simulink model "Velo"  (R2019a)
settings: Solver=ode45  StartTime=0  StopTime=4000  FixedStep=1e-3  MaxStep=0.01  RelTol=1e-3  EnableMultiTasking=on
InitFcn:
  | Initialisation
values from neighbouring files (symbols this model uses):
  assist =     [assit_lim.mat]
  cyclist =     [Cyclist_Profile.mat]
  env =     [Uvrier_HEI_Profile.mat]
undefined symbols (not defined in the file or in its folder): cycle
libraries: simulink x1
settings Model: ExtModeTrigMode=oneshot  ExtModeArmWhenConnect=off  Creator=Walter  LastModifiedBy=philippe.barrade
settings DataIOCC: SaveFormat=Array  SignalLoggingSaveFormat=ModelDataLogs  SaveOutput=off  SignalLogging=off  SaveTime=off  ReturnWorkspaceOutputs=off  SignalLoggingName=sigsOut
settings OptimizationCC: BooleanDataType=off  ExpressionDepthLimit=2147483647  InitFltsAndDblsToZero=on  LifeSpan=inf
settings DebuggingCC: SaveWithParameterizedLinksMsg=none  UnderspecifiedInitializationDetection=Classic  MergeDetectMultiDrivingBlocksExec=none  SignalResolutionControl=TryResolveAllWithWarning  MultiTaskDSMMsg=warning  MultiTaskCondExecSysMsg=none  FcnCallInpInsideContextMsg=warning  StateNameClashWarn=warning  SFUnexpectedBacktrackingDiag=warning  SFNoUnconditionalDefaultTransitionDiag=warning  SFExecutionAtInitializationDiag=none  ArithmeticOperatorsInVariantConditions=warning
settings HardwareCC: ProdBitPerPointer=32  ProdBitPerSizeT=32  ProdBitPerPtrDiffT=32  ProdLargestAtomicFloat=None  ProdIntDivRoundTo=Undefined  ProdEndianess=Unspecified  ProdWordSize=32  ProdHWDeviceType=32-bit Generic  TargetUnknown=on
settings ModelReferenceCC: PropagateSignalLabelsOutOfModel=off
settings SFSimCC: SimUseLocalCustomCode=off
settings RTWCC: GenerateMakefile=off  RTWUseLocalCustomCode=off
settings CodeAppCC: StateflowObjectComments=on
settings GRTTargetCC: TargetLangStandard=C89/C90 (ANSI)  ModelReferenceCompliant=off  CompOptLevelCompliant=off  GeneratePreprocessorConditionals=Disable all  CombineOutputUpdateFcns=off  MatFileLogging=off  GRTInterface=on
settings ConfigComp: CovMetricSettings=dw  CovHtmlReporting=on  CovSaveCumulativeToWorkspaceVar=on  CovSaveSingleToWorkspaceVar=on  CovExternalEMLEnable=off  CovSFcnEnable=off

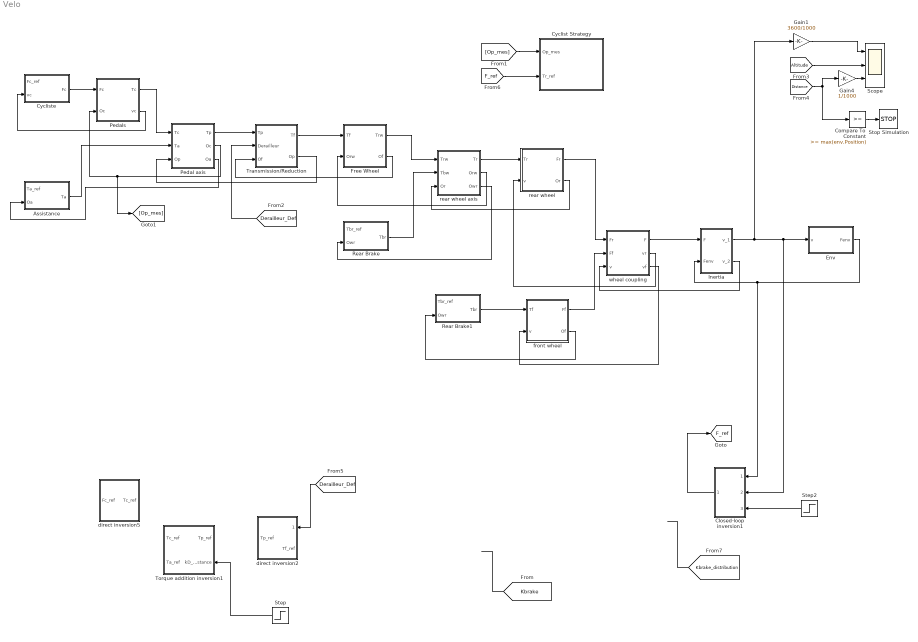
== system Velo ==
  Assistance : Subsystem
      mask Display:
      | plot(0,0,100,100, 1.2*[50,57.68,60.77,63.08,64.97,66.58,68,69.26,70.4, 	71.42,72.36,78.28,80,78.28,72.36,71.42,70.4, 	69.26,68,66.58,64.97,63.08,60.77,57.68,50,42.32, 	39.23,36.92,35.03,33.42,32,30.74,29.6,28.58, 	27.64,21.72,20,21.72,27.64,28.58,29.6,30.74,32, 	33.42,35.03,36.92,39.23,42.32,50]-10, 1.2*[20,21,22,23,24,25,26,27,28,29,30,40,50,60,70,71,72, 	73,74,75,76,77,78,79,80,79,78,77,76,75,74,73,72, 	71,70,60,50,40,30,29,28,27,26,25,24,23,22,21,20]-10)
      | disp('MS')
  Closed-loop inversion1 : Subsystem
      mask Display: plot(0,0,100,100, [10,30,90,70,10,90],[90,10,10,90,90,10])
  Compare To Constant : simulink/Logic and Bit Operations/Compare To Constant  relop=>=  const=max(env.Position)  OutDataTypeStr=boolean
  Cyclist Strategy : Subsystem
      mask Display:
      | color('white');
      | plot(0,0,100,100,[10,30,90,70,10], [90,10,10,90,90]);
  Cycliste : Subsystem
      mask Display:
      | plot(0,0,100,100, 1.2*[50,57.68,60.77,63.08,64.97,66.58,68,69.26,70.4, 	71.42,72.36,78.28,80,78.28,72.36,71.42,70.4, 	69.26,68,66.58,64.97,63.08,60.77,57.68,50,42.32, 	39.23,36.92,35.03,33.42,32,30.74,29.6,28.58, 	27.64,21.72,20,21.72,27.64,28.58,29.6,30.74,32, 	33.42,35.03,36.92,39.23,42.32,50]-10, 1.2*[20,21,22,23,24,25,26,27,28,29,30,40,50,60,70,71,72, 	73,74,75,76,77,78,79,80,79,78,77,76,75,74,73,72, 	71,70,60,50,40,30,29,28,27,26,25,24,23,22,21,20]-10)
      | disp('MS')
  Env : Subsystem
      mask Display:
      | plot(0,0,100,100, 1.2*[50,57.68,60.77,63.08,64.97,66.58,68,69.26,70.4, 	71.42,72.36,78.28,80,78.28,72.36,71.42,70.4, 	69.26,68,66.58,64.97,63.08,60.77,57.68,50,42.32, 	39.23,36.92,35.03,33.42,32,30.74,29.6,28.58, 	27.64,21.72,20,21.72,27.64,28.58,29.6,30.74,32, 	33.42,35.03,36.92,39.23,42.32,50]-10, 1.2*[20,21,22,23,24,25,26,27,28,29,30,40,50,60,70,71,72, 	73,74,75,76,77,78,79,80,79,78,77,76,75,74,73,72, 	71,70,60,50,40,30,29,28,27,26,25,24,23,22,21,20]-10)
      | disp('MS')
  Free Wheel : Subsystem  mask(Hacheur){}
      mask Display: plot(0,0,100,100,[10,10,90,90,10],[90,10,10,90,90])
  Gain1 : Gain  Gain=3600/1000
  Gain4 : Gain  Gain=1/1000
  Inertia : Subsystem  mask(CM){}
      mask Display: plot(0,0,100,100,[10,10,90,90,10],[90,10,10,90,90], [10,90],[10,90])
  Pedal axis : Subsystem  mask(CM){}
      mask Display: plot(0,0,100,100,[35,35,95,95,35],[65,10,10,65,65], [5,5,65,65,5],[90,35,35,90,90])
  Pedals : Subsystem  mask(Hacheur){}
      mask Display: plot(0,0,100,100,[10,10,90,90,10],[90,10,10,90,90])
  Rear Brake : Subsystem
      mask Display:
      | plot(0,0,100,100, 1.2*[50,57.68,60.77,63.08,64.97,66.58,68,69.26,70.4, 	71.42,72.36,78.28,80,78.28,72.36,71.42,70.4, 	69.26,68,66.58,64.97,63.08,60.77,57.68,50,42.32, 	39.23,36.92,35.03,33.42,32,30.74,29.6,28.58, 	27.64,21.72,20,21.72,27.64,28.58,29.6,30.74,32, 	33.42,35.03,36.92,39.23,42.32,50]-10, 1.2*[20,21,22,23,24,25,26,27,28,29,30,40,50,60,70,71,72, 	73,74,75,76,77,78,79,80,79,78,77,76,75,74,73,72, 	71,70,60,50,40,30,29,28,27,26,25,24,23,22,21,20]-10)
      | disp('MS')
  Rear Brake1 : Subsystem
      mask Display:
      | plot(0,0,100,100, 1.2*[50,57.68,60.77,63.08,64.97,66.58,68,69.26,70.4, 	71.42,72.36,78.28,80,78.28,72.36,71.42,70.4, 	69.26,68,66.58,64.97,63.08,60.77,57.68,50,42.32, 	39.23,36.92,35.03,33.42,32,30.74,29.6,28.58, 	27.64,21.72,20,21.72,27.64,28.58,29.6,30.74,32, 	33.42,35.03,36.92,39.23,42.32,50]-10, 1.2*[20,21,22,23,24,25,26,27,28,29,30,40,50,60,70,71,72, 	73,74,75,76,77,78,79,80,79,78,77,76,75,74,73,72, 	71,70,60,50,40,30,29,28,27,26,25,24,23,22,21,20]-10)
      | disp('MS')
  Scope : Scope  NumInputPorts=3
  Step : Step  Time=800  After=0.25  SampleTime=0
  Step2 : Step  Time=5.0  Before=0/3600  After=15000/3600  SampleTime=0
  Stop Simulation : Stop
  Torque addition inversion1 : Subsystem
      mask Display: plot(0,0,100,100,[20,40,100,80,20],[75,20,20,75,75], [0,20,80,60,0],[85,30,30,85,85])
  Transmission/Reduction : Subsystem  mask(Hacheur){}
      mask Display: plot(0,0,100,100,[10,10,90,90,10],[90,10,10,90,90])
  direct inversion2 : Subsystem
      mask Display: plot(0,0,100,100,[10,30,90,70,10],[90,10,10,90,90])
  direct inversion5 : Subsystem
      mask Display: plot(0,0,100,100,[10,30,90,70,10],[90,10,10,90,90])
  front wheel : Subsystem  mask(Hacheur){}
      mask Display: plot(0,0,100,100,[10,10,90,90,10],[90,10,10,90,90])
  rear wheel : Subsystem  mask(Hacheur){}
      mask Display: plot(0,0,100,100,[10,10,90,90,10],[90,10,10,90,90])
  rear wheel axis : Subsystem  mask(CM){}
      mask Display: plot(0,0,100,100,[35,35,95,95,35],[65,10,10,65,65], [5,5,65,65,5],[90,35,35,90,90])
  "wheel coupling " : Subsystem  mask(CM){}
      mask Display: plot(0,0,100,100,[35,35,95,95,35],[65,10,10,65,65], [5,5,65,65,5],[90,35,35,90,90])
  tag scope: F_ref=global
  wires:
  Inertia/1(v_1) -> Gain1/1, Closed-loop inversion1/2(V_mes), Env/1(v)
  Gain1/1 -> Scope/1
  [Altitude] -> Scope/2
  [Distance] -> Compare To Constant/1, Gain4/1
  Gain4/1 -> Scope/3
  [Op_mes] -> Cyclist Strategy/1(Op_mes)
  [F_ref] -> Cyclist Strategy/2(Tr_ref)
  Step/1 -> Torque addition inversion1/2(kD_assistance)
  Compare To Constant/1 -> Stop Simulation/1
  Step2/1 -> Closed-loop inversion1/3(V_ref)
  Cycliste/1(Fc) -> Pedals/1(Fc)
  Pedals/1(Tc) -> Pedal axis/1(Tc)
  Assistance/1(Ta) -> Pedal axis/2(Ta)
  Pedals/2(vc) -> Cycliste/2(vc)
  Pedal axis/2(Oc) -> [Op_mes], Pedals/2(Oc)
  Pedal axis/3(Oa) -> Assistance/2(Oa)
  Pedal axis/1(Tp) -> Transmission/Reduction/1(Tp)
  Transmission/Reduction/1(Tf) -> Free Wheel/1(Tf)
  Free Wheel/1(Trw) -> rear wheel axis/1(Trw)
  Rear Brake/1(Tbr) -> rear wheel axis/2(Tbw)
  Transmission/Reduction/2(Op) -> Pedal axis/3(Op)
  Free Wheel/2(Of) -> Transmission/Reduction/3(Of)
  rear wheel axis/2(Orw) -> Free Wheel/2(Orw)
  rear wheel axis/3(Owr) -> Rear Brake/2(Owr)
  rear wheel axis/1(Tr) -> rear wheel/1(Tr)
  Rear Brake1/1(Tbr) -> front wheel/1(Tf)
  front wheel/2(Of) -> Rear Brake1/2(Owr)
  rear wheel/1(Fr) -> "wheel coupling "/1(Fr)
  front wheel/1(Ff) -> "wheel coupling "/2(Ff)
  "wheel coupling "/2(vr) -> rear wheel/2(v)
  "wheel coupling "/3(vf) -> front wheel/2(v)
  "wheel coupling "/1(F) -> Inertia/1(F)
  Inertia/2(v_2) -> "wheel coupling "/3(v)
  Env/1(Fenv) -> Closed-loop inversion1/1(F_res), Inertia/2(Fenv)
  rear wheel/2(Or) -> rear wheel axis/3(Or)
  Closed-loop inversion1/1(Fr_ref) -> [F_ref]
  [Derailleur_Def] -> Transmission/Reduction/2(Derailleur)
  [Derailleur_Def] -> direct inversion2/1(Derailleur)
  [Kbrake] -> ?
  [Kbrake_distribution] -> ?
  ? -> Cycliste/1(Fc_ref)
  ? -> Assistance/1(Ta_ref)
  ? -> Rear Brake1/1(Tbr_ref)
  ? -> Rear Brake/1(Tbr_ref)

== system Velo/Assistance ==
  Ta_ref : Inport
  Oa : Inport  Port=2
  Memory : Memory
  MinMax : MinMax  Inputs=2
  Ta_lim : Lookup_n-D  NumberOfTableDimensions=1  BreakpointsForDimension1=assist.Op_ref  Table=assist.Ta_lim  InternalRulePriority=Speed  RndMeth=Simplest  InputSameDT=on
  Ta : Outport  InitialOutput=0
  wires:
  Oa/1 -> Memory/1
  Memory/1 -> Ta_lim/1
  MinMax/1 -> Ta/1
  Ta_ref/1 -> MinMax/1
  Ta_lim/1 -> MinMax/2

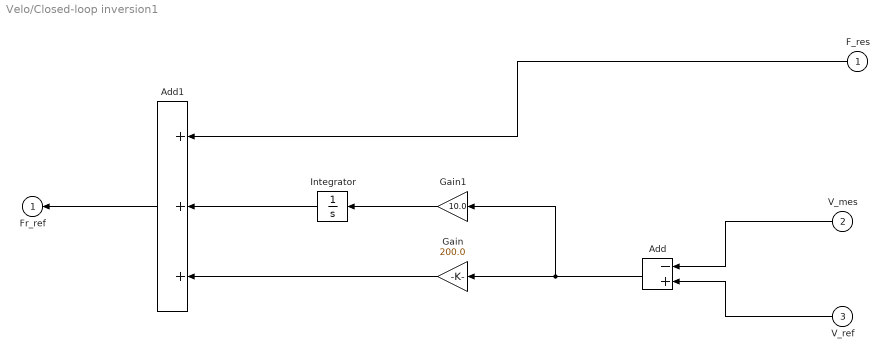
== system Velo/Closed-loop inversion1 ==
  F_res : Inport
  V_mes : Inport  Port=2
  V_ref : Inport  Port=3
  Add : Sum  Inputs=-+
  Add1 : Sum  Inputs=+++
  Gain : Gain  Gain=200.0
  Gain1 : Gain  Gain=10.0
  Integrator : Integrator  LimitOutput=on  UpperSaturationLimit=50  LowerSaturationLimit=-50
  Fr_ref : Outport  InitialOutput=0
  wires:
  V_mes/1 -> Add/1
  Gain1/1 -> Integrator/1
  Add/1 -> Gain1/1, Gain/1
  Add1/1 -> Fr_ref/1
  V_ref/1 -> Add/2
  Gain/1 -> Add1/3
  Integrator/1 -> Add1/2
  F_res/1 -> Add1/1

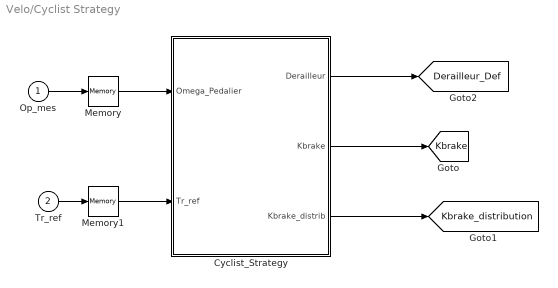
== system Velo/Cyclist Strategy ==
  Op_mes : Inport
  Tr_ref : Inport  Port=2
  Cyclist_Strategy : MATLAB Function  TreatAsAtomicUnit=on
  Memory : Memory
  Memory1 : Memory
  tag scope: Derailleur_Def=global, Kbrake=global, Kbrake_distribution=global
  wires:
  Op_mes/1 -> Memory/1
  Cyclist_Strategy/1(Derailleur) -> [Derailleur_Def]
  Memory/1 -> Cyclist_Strategy/1(Omega_Pedalier)
  Tr_ref/1 -> Memory1/1
  Memory1/1 -> Cyclist_Strategy/2(Tr_ref)
  Cyclist_Strategy/2(Kbrake) -> [Kbrake]
  Cyclist_Strategy/3(Kbrake_distrib) -> [Kbrake_distribution]

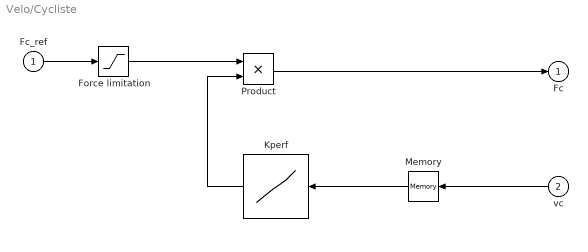
== system Velo/Cycliste ==
  Fc_ref : Inport
  vc : Inport  Port=2
  Force limitation : Saturate  UpperLimit=cyclist.Fc_max
  Kperf : Lookup_n-D  NumberOfTableDimensions=1  BreakpointsForDimension1=cyclist.Vref_ms  Table=cyclist.Kperf  InternalRulePriority=Speed  RndMeth=Simplest  InputSameDT=on
  Memory : Memory
  Product : Product
  Fc : Outport  InitialOutput=0
  wires:
  vc/1 -> Memory/1
  Memory/1 -> Kperf/1
  Product/1 -> Fc/1
  Fc_ref/1 -> Force limitation/1
  Kperf/1 -> Product/2
  Force limitation/1 -> Product/1

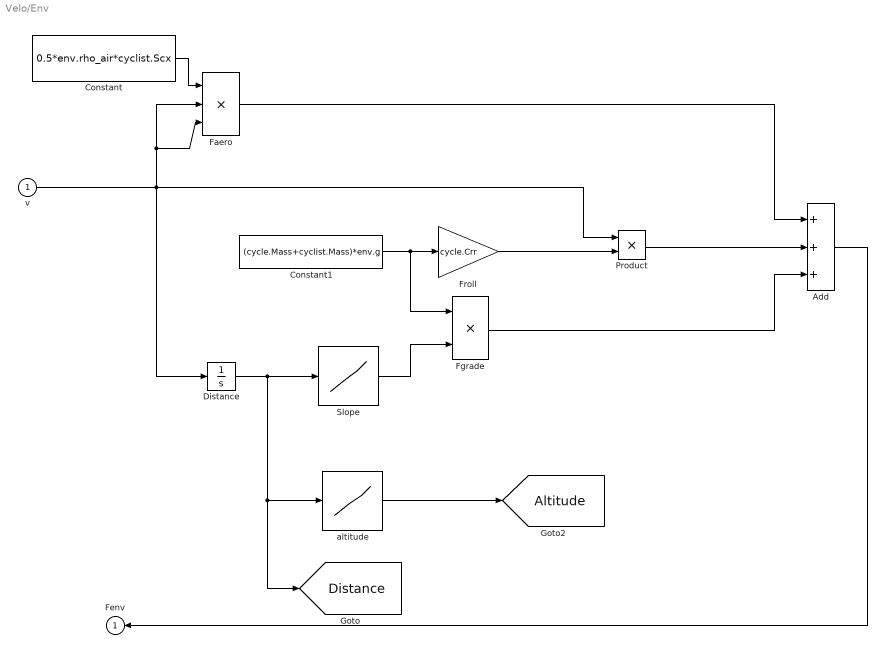
== system Velo/Env ==
  v : Inport
  Add : Sum  Inputs=+++
  Constant : Constant  Value=0.5*env.rho_air*cyclist.Scx
  Constant1 : Constant  Value=(cycle.Mass+cyclist.Mass)*env.g
  Distance : Integrator
  Faero : Product  Inputs=3  RndMeth=Zero
  Fgrade : Product  RndMeth=Zero
  Froll : Gain  Gain=cycle.Crr
  Product : Product  RndMeth=Zero
  Slope : Lookup  InputValues=env.Position  Table=env.Slope  LookUpMeth=Interpolation-Use End Values
  altitude : Lookup  InputValues=env.Position  Table=env.Altitude  LookUpMeth=Interpolation-Use End Values
  Fenv : Outport  InitialOutput=0
  tag scope: Altitude=global, Distance=global
  wires:
  Constant1/1 -> Froll/1, Fgrade/1
  Distance/1 -> [Distance], altitude/1, Slope/1
  Slope/1 -> Fgrade/2
  Faero/1 -> Add/1
  Fgrade/1 -> Add/3
  Add/1 -> Fenv/1
  Product/1 -> Add/2
  Froll/1 -> Product/2
  Constant/1 -> Faero/1
  v/1 -> Product/1, Distance/1, Faero/2, Faero/3
  altitude/1 -> [Altitude]

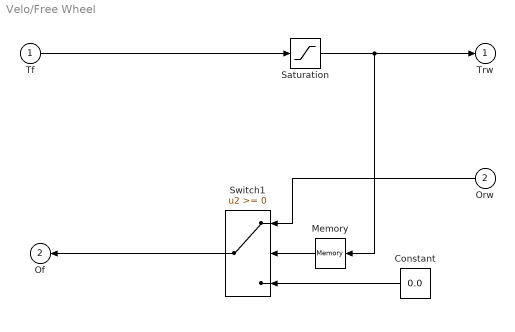
== system Velo/Free Wheel ==
  Tf : Inport
  Orw : Inport  Port=2
  Constant : Constant  Value=0.0
  Memory : Memory
  Saturation : Saturate  UpperLimit=Inf  LowerLimit=-1e-6
  Switch1 : Switch
  Trw : Outport  InitialOutput=0
  Of : Outport  Port=2  InitialOutput=0
  wires:
  Tf/1 -> Saturation/1
  Saturation/1 -> Trw/1, Memory/1
  Orw/1 -> Switch1/1
  Switch1/1 -> Of/1
  Constant/1 -> Switch1/3
  Memory/1 -> Switch1/2

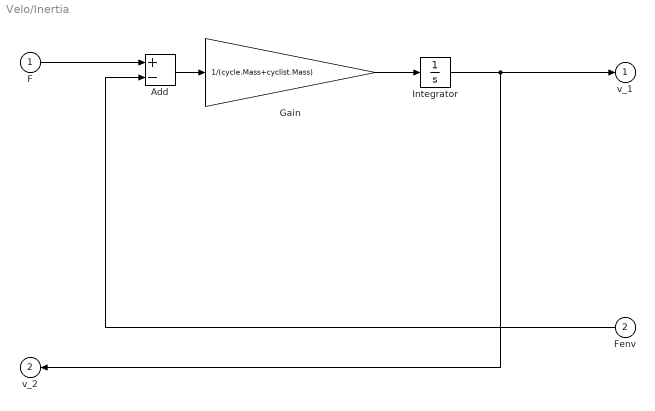
== system Velo/Inertia ==
  F : Inport
  Fenv : Inport  Port=2
  Add : Sum  Inputs=+-
  Gain : Gain  Gain=1/(cycle.Mass+cyclist.Mass)
  Integrator : Integrator
  v_1 : Outport  InitialOutput=0
  v_2 : Outport  Port=2  InitialOutput=0
  wires:
  F/1 -> Add/1
  Fenv/1 -> Add/2
  Add/1 -> Gain/1
  Gain/1 -> Integrator/1
  Integrator/1 -> v_1/1, v_2/1

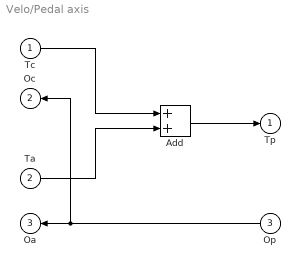
== system Velo/Pedal axis ==
  Tc : Inport
  Ta : Inport  Port=2
  Op : Inport  Port=3
  Add : Sum
  Tp : Outport  InitialOutput=0
  Oc : Outport  Port=2  InitialOutput=0
  Oa : Outport  Port=3  InitialOutput=0
  wires:
  Add/1 -> Tp/1
  Tc/1 -> Add/1
  Ta/1 -> Add/2
  Op/1 -> Oa/1, Oc/1

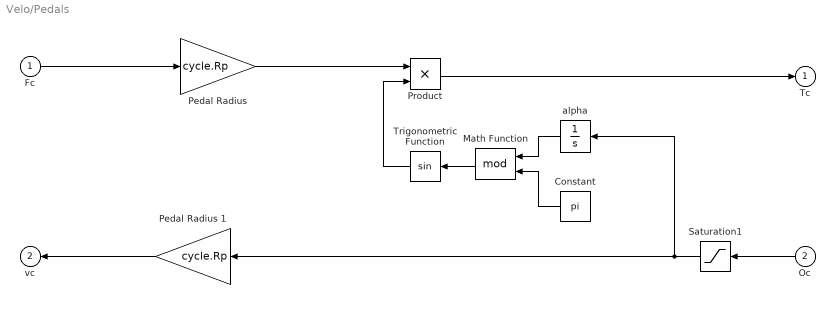
== system Velo/Pedals ==
  Fc : Inport
  Oc : Inport  Port=2
  Constant : Constant  Value=pi
  Math Function : Math  Operator=mod  SaturateOnIntegerOverflow=on
  Pedal Radius : Gain  Gain=cycle.Rp
  Pedal Radius 1 : Gain  Gain=cycle.Rp
  Product : Product
  Saturation1 : Saturate  UpperLimit=Inf  LowerLimit=1e-3
  Trigonometric Function : Trigonometry
  alpha : Integrator  InitialCondition=pi/2
  Tc : Outport  InitialOutput=0
  vc : Outport  Port=2  InitialOutput=0
  wires:
  Oc/1 -> Saturation1/1
  Trigonometric Function/1 -> Product/2
  Product/1 -> Tc/1
  Math Function/1 -> Trigonometric Function/1
  alpha/1 -> Math Function/1
  Constant/1 -> Math Function/2
  Saturation1/1 -> Pedal Radius 1/1, alpha/1
  Fc/1 -> Pedal Radius/1
  Pedal Radius 1/1 -> vc/1
  Pedal Radius/1 -> Product/1

== system Velo/Rear Brake ==
  Tbr_ref : Inport
  Owr : Inport  Port=2
  Saturation : Saturate  UpperLimit=0  LowerLimit=-1e3
  Terminator : Terminator
  Tbr : Outport  InitialOutput=0
  wires:
  Tbr_ref/1 -> Saturation/1
  Saturation/1 -> Tbr/1
  Owr/1 -> Terminator/1

== system Velo/Rear Brake1 ==
  Tbr_ref : Inport
  Owr : Inport  Port=2
  Saturation : Saturate  UpperLimit=0  LowerLimit=-1e3
  Terminator : Terminator
  Tbr : Outport  InitialOutput=0
  wires:
  Tbr_ref/1 -> Saturation/1
  Saturation/1 -> Tbr/1
  Owr/1 -> Terminator/1

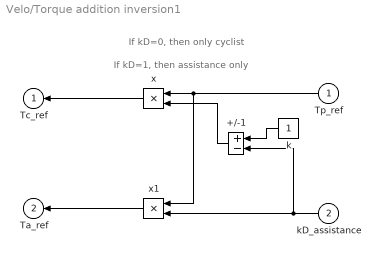
== system Velo/Torque addition inversion1 ==
  note: If kD=0, then only cyclist
  note: If kD=1, then assistance only
  Tp_ref : Inport
  kD_assistance : Inport  Port=2
  +/-1 : Sum  Inputs=+-  SaturateOnIntegerOverflow=on  InputSameDT=on  OutDataTypeStr=Inherit: Same as first input
  k : Constant
  x : Product  SaturateOnIntegerOverflow=on  InputSameDT=on  OutDataTypeStr=Inherit: Same as first input
  x1 : Product  SaturateOnIntegerOverflow=on  InputSameDT=on  OutDataTypeStr=Inherit: Same as first input
  Tc_ref : Outport  InitialOutput=0
  Ta_ref : Outport  Port=2  InitialOutput=0
  wires:
  Tp_ref/1 -> x1/1, x/1
  x1/1 -> Ta_ref/1
  x/1 -> Tc_ref/1
  k/1 -> +/-1/1
  kD_assistance/1 -> x1/2, +/-1/2
  +/-1/1 -> x/2

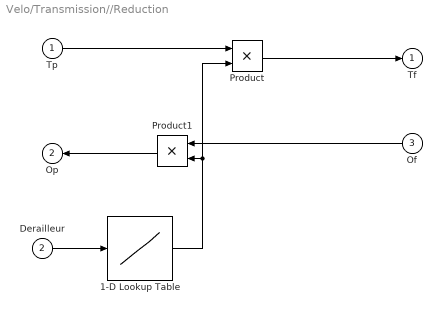
== system Velo/Transmission//Reduction ==
  Tp : Inport
  Derailleur : Inport  Port=2
  Of : Inport  Port=3
  1-D Lookup Table : Lookup_n-D  NumberOfTableDimensions=1  BreakpointsForDimension1=1:1:10  Table=cycle.Speed  InternalRulePriority=Speed  RndMeth=Simplest  InputSameDT=on
  Product : Product  RndMeth=Zero
  Product1 : Product  RndMeth=Zero
  Tf : Outport  InitialOutput=0
  Op : Outport  Port=2  InitialOutput=0
  wires:
  Tp/1 -> Product/1
  Product/1 -> Tf/1
  Product1/1 -> Op/1
  Of/1 -> Product1/1
  Derailleur/1 -> 1-D Lookup Table/1
  1-D Lookup Table/1 -> Product/2, Product1/2

== system Velo/direct inversion2 ==
  Derailleur : Inport
  Tf_ref : Inport  Port=2
  1-D Lookup Table : Lookup_n-D  NumberOfTableDimensions=1  BreakpointsForDimension1=1:1:10  Table=cycle.Speed  InternalRulePriority=Speed  RndMeth=Simplest  InputSameDT=on
  Product : Product  Inputs=*/  RndMeth=Zero
  Tp_ref : Outport  InitialOutput=0
  wires:
  Tf_ref/1 -> Product/1
  Derailleur/1 -> 1-D Lookup Table/1
  1-D Lookup Table/1 -> Product/2
  Product/1 -> Tp_ref/1

== system Velo/direct inversion5 ==
  Tc_ref : Inport
  Pedal Radius : Gain  Gain=1/cycle.Rp
  Fc_ref : Outport  InitialOutput=0
  wires:
  Tc_ref/1 -> Pedal Radius/1
  Pedal Radius/1 -> Fc_ref/1

== system Velo/front wheel ==
  Tf : Inport
  v : Inport  Port=2
  Gain : Gain  Gain=1/cycle.Rw
  Gain1 : Gain  Gain=1/cycle.Rw
  Ff : Outport  InitialOutput=0
  Of : Outport  Port=2  InitialOutput=0
  wires:
  Gain/1 -> Ff/1
  Tf/1 -> Gain/1
  v/1 -> Gain1/1
  Gain1/1 -> Of/1

== system Velo/rear wheel ==
  Tr : Inport
  v : Inport  Port=2
  Gain : Gain  Gain=1/cycle.Rw
  Gain1 : Gain  Gain=1/cycle.Rw
  Fr : Outport  InitialOutput=0
  Or : Outport  Port=2  InitialOutput=0
  wires:
  Gain/1 -> Fr/1
  Tr/1 -> Gain/1
  v/1 -> Gain1/1
  Gain1/1 -> Or/1

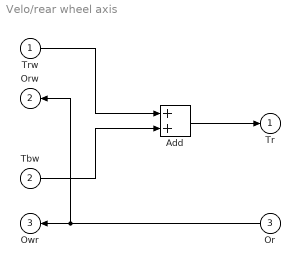
== system Velo/rear wheel axis ==
  Trw : Inport
  Tbw : Inport  Port=2
  Or : Inport  Port=3
  Add : Sum
  Tr : Outport  InitialOutput=0
  Orw : Outport  Port=2  InitialOutput=0
  Owr : Outport  Port=3  InitialOutput=0
  wires:
  Add/1 -> Tr/1
  Trw/1 -> Add/1
  Tbw/1 -> Add/2
  Or/1 -> Owr/1, Orw/1

== system Velo/wheel coupling  ==
  Fr : Inport
  Ff : Inport  Port=2
  v : Inport  Port=3
  Add : Sum
  F : Outport  InitialOutput=0
  vr : Outport  Port=2  InitialOutput=0
  vf : Outport  Port=3  InitialOutput=0
  wires:
  Add/1 -> F/1
  Fr/1 -> Add/1
  Ff/1 -> Add/2
  v/1 -> vf/1, vr/1

== matlab function Velo/Cyclist Strategy/Cyclist_Strategy ==
  data: Omega_Pedalier input; Derailleur output; Tr_ref input; Kbrake output; Kbrake_distrib output
function [Derailleur,Kbrake,Kbrake_distrib] = fcn(Omega_Pedalier,Tr_ref)

persistent Derailleur_ref

if isempty(Derailleur_ref)
    Derailleur_ref = 1;
end

%% Speed management
N_pedalier = Omega_Pedalier/2/pi;
if N_pedalier>1.6
    Derailleur = Derailleur_ref+1;
else
    if N_pedalier<0.8
        Derailleur = Derailleur_ref-1;
    else
        Derailleur = Derailleur_ref;
    end
end

Derailleur = min(Derailleur,10);
Derailleur = max(Derailleur,1);
Derailleur_ref = Derailleur;

%% Brake management
if Tr_ref<0
    Kbrake = 1.0;
    Kbrake_distrib = 0.25;
else
    Kbrake = 0.0;
    Kbrake_distrib = 1.0;
end
